simulink model "ramadan_2021"  (R2020a)
settings: Solver=ode15s  StartTime=0.0  StopTime=20  MaxStep=1e-2  MinStep=1e-20  RelTol=1e-3
StartFcn:
  | tic
StopFcn:
  | toc
  | 
  | 
  | %if GimbalLockFlag
  |  % fprintf(2, 'Almost reached Gimbal Lock of IMU. Simulation stopped.\n')
  | %end
  | 
  | %fprintf('Elapsed time: %4.2f sec (%4.2f%% realtime)\n', a, tout(end)/a*100)
values from neighbouring files (symbols this model uses):
  Balance02 = param(28:31)    [assign_parameters.m]
  Balance13 = param(32:35)    [assign_parameters.m]
  BalanceTrunk = param(22:23)    [assign_parameters.m]
  BalanceTrunkLat = param(24:27)    [assign_parameters.m]
  BasisStim = param(1:11)    [assign_parameters.m]
  CompliantLeg = param(12:14)    [assign_parameters.m]
  CompliantLegLat = param(15)    [assign_parameters.m]
  PreventKneeOverextension = param(16:21)    [assign_parameters.m]
  propulsion = dataset(i,3)    [AssignDataset_BasisPoints.m]    (also in assign_parameters.m = param(43))
  stepDur = dataset(i,2)    [AssignDataset_BasisPoints.m]    (also in assign_parameters.m = param(44))
  Target02 = dataset(i,8:10)    [AssignDataset_BasisPoints.m]    (also in assign_parameters.m = param(36:38))
  Target13 = dataset(i,5:7)    [AssignDataset_BasisPoints.m]    (also in assign_parameters.m = param(39:41))
  Target_lat = param(45)    [assign_parameters.m]
  theta0 = dataset(i,4)    [AssignDataset_BasisPoints.m]    (also in assign_parameters.m = param(42))
  v_init = dataset(i,1)    [AssignDataset_BasisPoints.m]    (also in assign_parameters.m = 1.25)
  WramameiSL_1000 = readmatrix('WSL_1000_Norm_Sigmoid_MSE_cont.csv')    [nms3D_prep.m]
  ZramameiSL_1000 = readmatrix('ZSL_1000_Norm_Sigmoid_MSE_cont.csv')    [nms3D_prep.m]
undefined symbols (not defined in the file or in its folder): ICs, mParams, X, Y, Z
libraries: nesl_utility x110, sm_lib x88, simulink x81, eeGeneralControl x30, robotmaniplib x10, dspinverses x9, robotcorelib x5, dspmathops x3, vrlib x1
(part 7 of 8)

== system ramadan_2021/Muscle Actuation Layer/Muscles Right/Muscle Dynamics (Vectorized)/CE inverse force-velocity relation ==
  note: CE Inverse Force-Velocity Relationship
  Fv[Fmax] : Inport
  1 : Product  Inputs=/*
  Constant{1,3..4,8} (4 alike) : Constant
  Constant2 : Constant  Value=mParams.muscles.N
  Curvature : Gain  Gain=mParams.muscles.K  SaturateOnIntegerOverflow=on  OutDataTypeStr=Inherit: Same as input  ParamDataTypeStr=Inherit: Same as input
  Curvature1 : Gain  Gain=7.56*mParams.muscles.K  SaturateOnIntegerOverflow=on  OutDataTypeStr=Inherit: Same as input  ParamDataTypeStr=Inherit: Same as input
  Logical Operator : Logic  Operator=NOT  AllPortsSameDT=off  OutDataTypeStr=boolean
  Logical Operator1 : Logic  Operator=NOT  AllPortsSameDT=off  OutDataTypeStr=boolean
  Slope : Gain  Gain=1e-2  SaturateOnIntegerOverflow=on  OutDataTypeStr=Inherit: Same as input  ParamDataTypeStr=Inherit: Same as input
  Sum1 : Sum  Inputs=|++  InputSameDT=on  SaturateOnIntegerOverflow=on  OutDataTypeStr=Inherit: Same as first input
  Sum2 : Sum  InputSameDT=on  SaturateOnIntegerOverflow=on  OutDataTypeStr=Inherit: Same as first input
  Sum3 : Sum  Inputs=++|  InputSameDT=on  SaturateOnIntegerOverflow=on  OutDataTypeStr=Inherit: Same as first input
  Sum4 : Sum  Inputs=|+-  InputSameDT=on  SaturateOnIntegerOverflow=on  OutDataTypeStr=Inherit: Same as first input
  Sum5 : Sum  Inputs=|-+  InputSameDT=on  SaturateOnIntegerOverflow=on  OutDataTypeStr=Inherit: Same as first input
  Sum6 : Sum  Inputs=-+|  InputSameDT=on  SaturateOnIntegerOverflow=on  OutDataTypeStr=Inherit: Same as first input
  Sum7 : Sum  Inputs=|++  InputSameDT=on  SaturateOnIntegerOverflow=on  OutDataTypeStr=Inherit: Same as first input
  Sum8 : Sum  Inputs=+-|  InputSameDT=on  SaturateOnIntegerOverflow=on  OutDataTypeStr=Inherit: Same as first input
  Sum9 : Sum  InputSameDT=on  SaturateOnIntegerOverflow=on  OutDataTypeStr=Inherit: Same as first input
  extension force within bound? : simulink/Logic and Bit Operations/Compare To Constant  relop=<=  const=mParams.muscles.N  OutDataTypeStr=boolean  ZeroCross=off
  force indicating contraction? : simulink/Logic and Bit Operations/Compare To Constant  relop=<=  const=1  OutDataTypeStr=boolean  ZeroCross=off
  v_concentric : Product  Inputs=*/
  v_concentric1 : Product  Inputs=**
  v_excentric <=N 1 : Product  Inputs=***
  v_excentric <N : Product  Inputs=*/
  v_excentric >N : Product  Inputs=**
  v[vmax] : Outport  VectorParamsAs1DForOutWhenUnconnected=off
  wires:
  Sum2/1 -> Sum9/2
  v_excentric <=N 1/1 -> Sum2/1
  Logical Operator1/1 -> v_excentric >N/1
  v_excentric >N/1 -> Sum2/2
  Logical Operator/1 -> v_excentric <=N 1/1
  Fv[Fmax]/1 -> extension force within bound?/1, force indicating contraction?/1, Curvature/1, Sum4/1, Sum6/2
  extension force within bound?/1 -> Logical Operator1/1, v_excentric <=N 1/3
  force indicating contraction?/1 -> Logical Operator/1, v_concentric1/2
  Sum1/1 -> v_excentric >N/2
  v_concentric1/1 -> Sum9/1
  v_excentric <N/1 -> v_excentric <=N 1/2
  Constant3/1 -> Sum5/1
  Sum5/1 -> 1/1
  Constant2/1 -> Sum5/2, Sum6/1
  Sum6/1 -> Slope/1, 1/2
  Constant8/1 -> Sum1/2
  Slope/1 -> Sum1/1
  Sum9/1 -> v[vmax]/1
  v_concentric/1 -> v_concentric1/1
  Sum7/1 -> v_excentric <N/1
  Sum8/1 -> v_excentric <N/2
  Curvature1/1 -> Sum8/2
  Constant4/1 -> Sum8/1, Sum7/2
  1/1 -> Curvature1/1, Sum7/1
  Sum3/1 -> v_concentric/2
  Sum4/1 -> v_concentric/1
  Constant1/1 -> Sum3/1, Sum4/2
  Curvature/1 -> Sum3/2

== system ramadan_2021/Muscle Actuation Layer/Muscles Right/Muscle Dynamics (Vectorized)/PE force-length relation ==
  note: Parallel Elasticity PE
  lce [lopt] : Inport
  Constant3 : Constant
  Math Function2 : Math  Operator=square  SignedPower=on  SaturateOnIntegerOverflow=on
  Sum1 : Sum  Inputs=|+-  InputSameDT=on  SaturateOnIntegerOverflow=on  OutDataTypeStr=Inherit: Same as first input
  force of buffer elasticity : Product  Inputs=**
  parallel elasticity engaged? : simulink/Logic and Bit Operations/Compare To Zero  relop=>  OutDataTypeStr=boolean  ZeroCross=off
  reference strain [lopt] : Constant  Value=mParams.muscles.w
  relative strain : Product  Inputs=*/
  fpe [Fmax] : Outport  VectorParamsAs1DForOutWhenUnconnected=off
  wires:
  parallel elasticity engaged?/1 -> force of buffer elasticity/1
  force of buffer elasticity/1 -> fpe [Fmax]/1
  Math Function2/1 -> force of buffer elasticity/2
  relative strain/1 -> Math Function2/1
  reference strain [lopt]/1 -> relative strain/2
  Sum1/1 -> relative strain/1, parallel elasticity engaged?/1
  Constant3/1 -> Sum1/2
  lce [lopt]/1 -> Sum1/1

== system ramadan_2021/Muscle Actuation Layer/Muscles Right/Muscle Dynamics (Vectorized)/SE force-length relation ==
  note: SE Force-Length Relationship
  lse [lslack] : Inport
  Constant1 : Constant
  Math Function : Math  Operator=square  SignedPower=on  SaturateOnIntegerOverflow=on
  Sum4 : Sum  Inputs=|+-  InputSameDT=on  SaturateOnIntegerOverflow=on  OutDataTypeStr=Inherit: Same as first input
  force above slack length : Product  Inputs=**
  greater than slack length? : simulink/Logic and Bit Operations/Compare To Zero  relop=>  OutDataTypeStr=boolean  ZeroCross=off
  reference strain [lslack] : Constant  Value=mParams.muscles.eref
  relative strain : Product  Inputs=*/
  fse [Fmax] : Outport  VectorParamsAs1DForOutWhenUnconnected=off
  wires:
  force above slack length/1 -> fse [Fmax]/1
  greater than slack length?/1 -> force above slack length/1
  Constant1/1 -> Sum4/2
  Sum4/1 -> relative strain/1, greater than slack length?/1
  relative strain/1 -> Math Function/1
  lse [lslack]/1 -> Sum4/1
  Math Function/1 -> force above slack length/2
  reference strain [lslack]/1 -> relative strain/2

== system ramadan_2021/Muscle Actuation Layer/Muscles Right/Muscle Torque Contributions/Subsystem ==
  F VAS : Inport
  Moment Arm VAS : Inport  Port=2
  F SOL : Inport  Port=3
  Moment Arm SOL : Inport  Port=4
  Constant : Constant  Value=mParams.muscles.FmaxVec(7)
  Constant1 : Constant  Value=mParams.muscles.FmaxVec(10)
  Divide2 : Product  Inputs=*/
  Product{7..8,11..12} (4 alike) : Product
  Sum4 : Sum
  Sum6 : Sum
  "Leg Torque " : Outport
  wires:
  Sum4/1 -> Divide2/2
  Divide2/1 -> "Leg Torque "/1
  Moment Arm SOL/1 -> Product7/1, Product11/2
  Product11/1 -> Sum6/2
  Constant/1 -> Product8/2
  F VAS/1 -> Product12/1
  Moment Arm VAS/1 -> Product8/1, Product12/2
  Product7/1 -> Sum4/2
  F SOL/1 -> Product11/1
  Sum6/1 -> Divide2/1
  Product12/1 -> Sum6/1
  Constant1/1 -> Product7/2
  Product8/1 -> Sum4/1

== system ramadan_2021/Supraspinal Level/Subsystem/Compute positives forces that generate desired torque profiles/Left ==
  Desired Torques : Inport
  Angles : Inport  Port=2
  Constant : Constant  Value=WramameiSL_1000  VectorParams1D=off  SampleTime=-1
  Constant1 : Constant  Value=|
      | [1.666708374023437500e+01
      | -3.333266830444335938e+01]
  Constant2 : Constant  Value=ZramameiSL_1000
  Denorm : Gain  Gain=[2000, 1500, 3000, 1200, 6000, 350, 1500, 4000, 800]
  Matrix Concatenate : Concatenate  Mode=Multidimensional array
  Matrix Concatenate4 : Concatenate  Mode=Multidimensional array  ConcatenateDimension=2
  Matrix Multiply2 : Product  Multiplication=Matrix(*)
  Matrix Multiply3 : Product  Multiplication=Matrix(*)
  Matrix Multiply8 : Product  Multiplication=Matrix(*)
  Multiply : Gain  Gain=1/960
  Multiply2 : Gain  Gain=1/3.0543
  Saturation : Saturate  UpperLimit=inf  LowerLimit=0  ZeroCross=off
  Saturation2 : Saturate  UpperLimit=inf  LowerLimit=0  ZeroCross=off
  Selector : Selector  InputPortWidth=4  IndexOptions=Index vector (dialog)  Indices=[1 3 4]  OutputSizes=1
  Selector1 : Selector  InputPortWidth=4  IndexOptions=Index vector (dialog)  Indices=[3 4]  OutputSizes=1
  Selector8 : Selector  InputPortWidth=4  IndexOptions=Index vector (dialog)  Indices=2  OutputSizes=1
  Transpose3 : Math  Operator=transpose  SaturateOnIntegerOverflow=on
  Transpose9 : Math  Operator=transpose  SaturateOnIntegerOverflow=on
  sigmoid : Subsystem
  Forces : Outport
  wires:
  Desired Torques/1 -> Selector/1, Selector8/1
  Selector1/1 -> Multiply2/1
  Matrix Multiply2/1 -> Saturation/1
  Selector/1 -> Multiply/1
  Constant/1 -> Matrix Multiply3/2
  Constant2/1 -> Matrix Multiply2/2
  Angles/1 -> Selector1/1
  Matrix Multiply8/1 -> Saturation2/1
  Constant1/1 -> Transpose9/1
  Selector8/1 -> Matrix Multiply8/1
  Transpose9/1 -> Matrix Multiply8/2
  Saturation/1 -> Denorm/1
  Matrix Concatenate4/1 -> Forces/1
  Saturation2/1 -> Matrix Concatenate4/1
  Transpose3/1 -> Matrix Multiply3/1
  Matrix Concatenate/1 -> Transpose3/1  "tr"
  Denorm/1 -> Matrix Concatenate4/2
  Multiply/1 -> Matrix Concatenate/1
  Multiply2/1 -> Matrix Concatenate/2
  sigmoid/1(Out1) -> Matrix Multiply2/1
  Matrix Multiply3/1 -> sigmoid/1(In1)

== system ramadan_2021/Supraspinal Level/Subsystem/Compute positives forces that generate desired torque profiles/Right ==
  Desired Torques : Inport
  Angles : Inport  Port=2
  Constant : Constant  Value=WramameiSL_1000  VectorParams1D=off  SampleTime=-1
  Constant1 : Constant  Value=|
      | [1.666708374023437500e+01
      | -3.333266830444335938e+01]
  Constant2 : Constant  Value=ZramameiSL_1000
  Denorm : Gain  Gain=[2000, 1500, 3000, 1200, 6000, 350, 1500, 4000, 800]
  Matrix Concatenate : Concatenate  Mode=Multidimensional array
  Matrix Concatenate4 : Concatenate  Mode=Multidimensional array  ConcatenateDimension=2
  Matrix Multiply2 : Product  Multiplication=Matrix(*)
  Matrix Multiply3 : Product  Multiplication=Matrix(*)
  Matrix Multiply8 : Product  Multiplication=Matrix(*)
  Multiply : Gain  Gain=1/960
  Multiply2 : Gain  Gain=1/3.0543
  Saturation : Saturate  UpperLimit=inf  LowerLimit=0  ZeroCross=off
  Saturation2 : Saturate  UpperLimit=inf  LowerLimit=0  ZeroCross=off
  Selector : Selector  InputPortWidth=4  IndexOptions=Index vector (dialog)  Indices=[1 3 4]  OutputSizes=1
  Selector1 : Selector  InputPortWidth=4  IndexOptions=Index vector (dialog)  Indices=[3 4]  OutputSizes=1
  Selector8 : Selector  InputPortWidth=4  IndexOptions=Index vector (dialog)  Indices=2  OutputSizes=1
  Transpose3 : Math  Operator=transpose  SaturateOnIntegerOverflow=on
  Transpose9 : Math  Operator=transpose  SaturateOnIntegerOverflow=on
  sigmoid : Subsystem
  Forces : Outport
  wires:
  Desired Torques/1 -> Selector/1, Selector8/1
  Selector1/1 -> Multiply2/1
  Matrix Multiply2/1 -> Saturation/1
  Selector/1 -> Multiply/1
  Constant/1 -> Matrix Multiply3/2
  Constant2/1 -> Matrix Multiply2/2
  Angles/1 -> Selector1/1
  Matrix Multiply8/1 -> Saturation2/1
  Constant1/1 -> Transpose9/1
  Selector8/1 -> Matrix Multiply8/1
  Transpose9/1 -> Matrix Multiply8/2
  Saturation/1 -> Denorm/1
  Matrix Concatenate4/1 -> Forces/1
  Saturation2/1 -> Matrix Concatenate4/1
  Transpose3/1 -> Matrix Multiply3/1
  Matrix Concatenate/1 -> Transpose3/1  "tr"
  Denorm/1 -> Matrix Concatenate4/2
  Multiply/1 -> Matrix Concatenate/1
  Multiply2/1 -> Matrix Concatenate/2
  sigmoid/1(Out1) -> Matrix Multiply2/1
  Matrix Multiply3/1 -> sigmoid/1(In1)

== system ramadan_2021/Supraspinal Level/Subsystem/Stance Leg2/Balance Control Equation [Ankle Strategy] ==
  Desired Acceleration (CoM) : Outport
  wires:
  [propulsion] -> Desired Acceleration (CoM)/1

== system ramadan_2021/Supraspinal Level/Subsystem/Stance Leg2/Stance Leg ==
  left/right : Inport
  Balance Control [Ankle Strategy] : Inport  Port=2
  Foot Orientation Left : Subsystem
  Foot Orientation Right : Subsystem
  Inverse Dynamics Left Leg : Subsystem
  Mux : Mux  Inputs=2
  Mux1 : Mux  Inputs=2
  NOT2 : Logic  Operator=NOT  AllPortsSameDT=off  OutDataTypeStr=boolean
  Selector : Selector  InputPortWidth=4  IndexOptions=Index vector (dialog)  Indices=[ 4 3 2 1]  OutputSizes=1
  Selector1 : Selector  InputPortWidth=4  IndexOptions=Index vector (dialog)  Indices=[ 4 3 2 1]  OutputSizes=1
  Subsystem : Subsystem
  Transpose : Math  Operator=transpose  SaturateOnIntegerOverflow=on
  long delay 1 : eeGeneralControl/Low-Pass Filter (Discrete or Continuous)  K=1  T=mParams.control.delays.long  B=inf  A=-inf  init_option=Inherited from block input  x0=0  Ts=0
  long delay 2 : eeGeneralControl/Low-Pass Filter (Discrete or Continuous)  K=1  T=mParams.control.delays.long  B=inf  A=-inf  init_option=Inherited from block input  x0=0  Ts=0
  long delay 4 : eeGeneralControl/Low-Pass Filter (Discrete or Continuous)  K=1  T=mParams.control.delays.long  B=inf  A=-inf  init_option=Inherited from block input  x0=0  Ts=0
  Push Off Left : Outport
  Push-Off Right : Outport  Port=2
  wires:
  [Rlegq] -> long delay 2/1
  Selector/1 -> Mux/2
  Selector1/1 -> Mux1/2
  [R_body] -> long delay 4/1
  left/right/1 -> NOT2/1, Inverse Dynamics Left Leg/2(left/right)
  Transpose/1 -> Foot Orientation Right/1(R Pelvis), Foot Orientation Left/1(R Pelvis)
  Foot Orientation Left/1(Orientation Foot (Z)) -> Mux1/1
  Foot Orientation Right/1(Foot Orientation (Z)) -> Mux/1
  Balance Control [Ankle Strategy]/1 -> Inverse Dynamics Left Leg/3(Task), Subsystem/3(Task)
  Inverse Dynamics Left Leg/1(Push-Off (Left)) -> Push Off Left/1
  Mux/1 -> Subsystem/1(Config [5])
  NOT2/1 -> Subsystem/2(left/right)
  Subsystem/1(Push-Off (Right)) -> Push-Off Right/1
  Mux1/1 -> Inverse Dynamics Left Leg/1(Config [5])
  long delay 1/1 -> Selector1/1
  long delay 2/1 -> Selector/1
  long delay 4/1 -> Transpose/1
  [Llegq] -> long delay 1/1

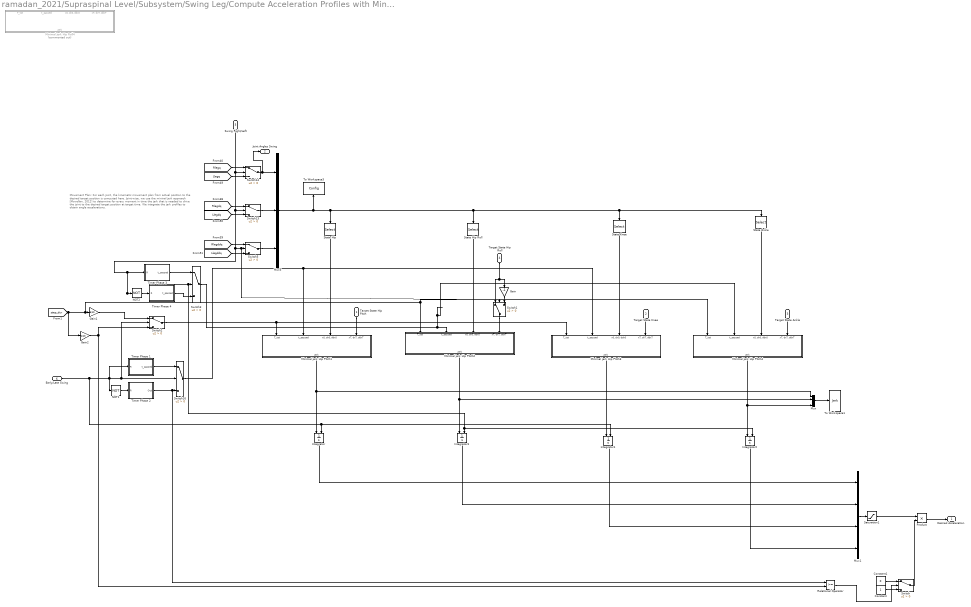
== system ramadan_2021/Supraspinal Level/Subsystem/Swing Leg/Compute Acceleration Profiles with Minimal Jerk Approach ==
  note: Movement Plan: For each joint, the kinematic movement plan from actual position to the desired target position is computed here. Joint-wise, we use the mininal jerk approach [Movellan, 2012] to determine for every moment in time the jerk that is needed to drive the joint to the desired target position at target time. We integrate the jerk profiles to obtain angle accelerations.
  Target State Hip Pitch : Inport
  Target State Knee : Inport  Port=2
  Target State Ankle : Inport  Port=3
  Target State Hip Roll : Inport  Port=4
  Swing Right/Left : Inport  Port=5
  Early/Late Swing : Inport  Port=6
  " Timer Phase 1" : Subsystem
  " Timer Phase 2" : Subsystem
  " Timer Phase 3" : Subsystem
  " Timer Phase 4" : Subsystem
  Constant : Constant
  Constant1 : Constant  Value=0
  Gain : Gain  Gain=-1
  Gain1 : Gain  Gain=6/10
  Gain2 : Gain  Gain=4/10
  Integrator{,1..3} (4 alike) : Integrator  ExternalReset=either  ZeroCross=off
  Minimal jerk Hip Pitch1 : Subsystem
  Minimal jerk Hip Pitch2 : Subsystem
  Minimal jerk Hip Pitch3 : Subsystem
  Minimal jerk Hip Pitch4 : Subsystem
  Minimal jerk Hip Roll4 : Subsystem  Commented=on
  Mux : Mux
  Mux1 : Mux
  Mux5 : Mux  Inputs=3
  NOT1 : Logic  Operator=NOT  AllPortsSameDT=off  OutDataTypeStr=boolean
  NOT2 : Logic  Operator=NOT  AllPortsSameDT=off  OutDataTypeStr=boolean
  Product : Product
  Relational Operator : RelationalOperator  OutDataTypeStr=boolean  ZeroCross=off  RndMeth=Simplest
  Saturation1 : Saturate  UpperLimit=2000  LowerLimit=-2000  ZeroCross=off
  State Ankle : Selector  InputPortWidth=12  IndexOptions=Index vector (dialog)  Indices=[4 8 12]  OutputSizes=1
  State Hip : Selector  InputPortWidth=12  IndexOptions=Index vector (dialog)  Indices=[1 5 9]  OutputSizes=1
  State Hip Roll : Selector  InputPortWidth=12  IndexOptions=Index vector (dialog)  Indices=[2 6 10 ]  OutputSizes=1
  State Knee : Selector  InputPortWidth=12  IndexOptions=Index vector (dialog)  Indices=[3 7 11 ]  OutputSizes=1
  Switch{,1..3,5,13..14,16} (8 alike) : Switch  Criteria=u2 > Threshold
  To Workspace1 : ToWorkspace  VariableName=Jerk  SampleTime=-1
      settings: Save2DSignal=2-D array (concatenate along first dimension)
  To Workspace3 : ToWorkspace  VariableName=Config  SampleTime=-1
      settings: Save2DSignal=2-D array (concatenate along first dimension)
  "Desired Acceleration " : Outport
  Joint Angles Swing : Outport  Port=2
  wires:
  State Hip/1 -> Minimal jerk Hip Pitch1/3("x0, dx0, ddx0")
  NOT1/1 -> " Timer Phase 2"/1(R)
  Mux1/1 -> Saturation1/1
  Switch2/1 -> Minimal jerk Hip Pitch1/1(T_tot), Minimal jerk Hip Pitch3/1(T_tot)
  [Llegddq] -> Switch5/3
  [Rlegq] -> Switch14/1
  [Llegdq] -> Switch13/3
  Target State Hip Pitch/1 -> Minimal jerk Hip Pitch1/4("xT, dxT, ddxT")
  Target State Knee/1 -> Minimal jerk Hip Pitch3/4("xT, dxT, ddxT")
  [Rlegddq] -> Switch5/1
  Integrator1/1 -> Mux1/3
  Switch5/1 -> Mux5/3
  [Llegq] -> Switch14/3
  State Knee/1 -> Minimal jerk Hip Pitch3/3("x0, dx0, ddx0")
  Target State Ankle/1 -> Minimal jerk Hip Pitch4/4("xT, dxT, ddxT")
  Integrator/1 -> Mux1/1
  Switch14/1 -> Joint Angles Swing/1, Mux5/1
  Integrator2/1 -> Mux1/4
  State Ankle/1 -> Minimal jerk Hip Pitch4/3("x0, dx0, ddx0")
  Switch13/1 -> Mux5/2
  [Rlegdq] -> Switch13/1
  Early/Late Swing/1 -> Switch2/2, Switch16/2, NOT1/1, " Timer Phase 1"/1(R), Integrator1/2, Integrator/2
  Swing Right/Left/1 -> Switch14/2, Switch13/2, Integrator2/2, Integrator3/2, Switch3/2, NOT2/1, " Timer Phase 3"/1(R), Switch1/2, Switch5/2
  Switch16/1 -> Minimal jerk Hip Pitch1/2(t_passed), Minimal jerk Hip Pitch3/2(t_passed)
  State Hip Roll/1 -> Minimal jerk Hip Pitch2/3("x0, dx0, ddx0")
  Integrator3/1 -> Mux1/2
  Switch1/1 -> Minimal jerk Hip Pitch2/4("xT, dxT, ddxT")
  Target State Hip Roll/1 -> Gain/1, Switch1/1
  Gain/1 -> Switch1/3
  [step_dur] -> Gain2/1, Minimal jerk Hip Pitch4/1(T_tot), Minimal jerk Hip Pitch2/1(T_tot), Gain1/1
  " Timer Phase 1"/1(t_passed) -> Switch16/1
  " Timer Phase 2"/1(Out) -> Relational Operator/1, Switch16/3
  Mux5/1 -> State Hip Roll/1, State Ankle/1, State Knee/1, State Hip/1, To Workspace3/1
  Mux/1 -> To Workspace1/1
  Minimal jerk Hip Pitch1/1(jerk) -> Mux/1, Integrator/1
  Minimal jerk Hip Pitch2/1(jerk) -> Mux/2, Integrator3/1
  Minimal jerk Hip Pitch3/1(jerk) -> Integrator1/1
  Minimal jerk Hip Pitch4/1(jerk) -> Mux/4, Integrator2/1
  Saturation1/1 -> Product/1
  Relational Operator/1 -> Switch/2
  Constant/1 -> Switch/3
  Constant1/1 -> Switch/1
  Switch/1 -> Product/2
  Product/1 -> "Desired Acceleration "/1
  Gain1/1 -> Switch2/1
  Gain2/1 -> Switch2/3, Relational Operator/2
  NOT2/1 -> " Timer Phase 4"/1(R)
  " Timer Phase 3"/1(t_passed) -> Switch3/1
  " Timer Phase 4"/1(t_passed) -> Switch3/3
  Switch3/1 -> Minimal jerk Hip Pitch4/2(t_passed), Minimal jerk Hip Pitch2/2(t_passed)

== system ramadan_2021/Supraspinal Level/Subsystem/Swing Leg/Compute Target States ==
  note: Target Joint States: Target joint angles, angle velocities and angle acceleration are defined here. For knee and ankle, values are constant. For hip pitch and hip roll, values are computed using the Balance Control mechanism from [Yin et. al. 2007].
      | Low pass filters are added here to compensate for abrupt changes in target angles at transitions between early and late swing.
  Left/Right : Inport
  Early/Late : Inport  Port=2
  Balance Control lateral : Subsystem
  Balance Control saggital : Subsystem
  Constant : Constant  Value=0
  Constant13 : Constant  Value=pi
  Gain3 : Gain  Gain=-1
  Low-Pass Filter (Discrete or Continuous)1 : eeGeneralControl/Low-Pass Filter (Discrete or Continuous)  K=1  T=0.1  B=inf  A=-inf  init_option=Inherited from block input  x0=-13  Ts=0
  Low-Pass Filter (Discrete or Continuous)2 : eeGeneralControl/Low-Pass Filter (Discrete or Continuous)  K=1  T=0.1  B=inf  A=-inf  init_option=Inherited from block input  x0=-13  Ts=0
  Minus1 : Sum
  Minus8 : Sum  Inputs=+++
  Mux{2..3,5..6} (4 alike) : Mux  Inputs=3
  Product : Product
  Sign : Signum  ZeroCross=off
  Hip Pitch Target : Outport
  Knee Target : Outport  Port=2
  Ankle Target : Outport  Port=3
  Hip Roll Target : Outport  Port=4
  wires:
  [TrunkRot_sag] -> Minus8/3
  Left/Right/1 -> Balance Control lateral/1(Left/Right), Balance Control saggital/1(Left/Right)
  Gain3/1 -> Minus8/1
  [swk] -> Mux5/1
  Balance Control lateral/1(theta_Hip_swing_target) -> Sign/1, Minus1/1
  Balance Control saggital/1(theta_Hip_swing_target) -> Gain3/1
  Mux5/1 -> Knee Target/1
  Constant13/1 -> Minus8/2
  [TrunkRot_lat] -> Minus1/2
  Mux2/1 -> Low-Pass Filter (Discrete or Continuous)2/1
  Mux6/1 -> Ankle Target/1
  Minus1/1 -> Mux2/1
  Low-Pass Filter (Discrete or Continuous)2/1 -> Hip Roll Target/1
  [swa] -> Mux6/1
  [swh_lat_a] -> Mux2/3
  [swh_lat_v] -> Product/1
  Product/1 -> Mux2/2
  Sign/1 -> Product/2
  Minus8/1 -> Mux3/1
  Mux3/1 -> Low-Pass Filter (Discrete or Continuous)1/1
  Low-Pass Filter (Discrete or Continuous)1/1 -> Hip Pitch Target/1
  Early/Late/1 -> Balance Control saggital/2(Early Late)
  Constant/1 -> Mux6/3, Mux6/2, Mux5/3, Mux3/2, Mux3/3, Mux5/2

== system ramadan_2021/Supraspinal Level/Subsystem/Swing Leg/Inverse Dynamics: Left Leg ==
  Desired Acceleration : Inport
  Enable : Inport  Port=2
  Inverse Dynamics : Subsystem
  Sensor Data from Body Layer : Subsystem
  Desired Torques : Outport
  Interaction Wrench : Outport  Port=2
  wires:
  Inverse Dynamics/1(" Desired Torques") -> Desired Torques/1
  Desired Acceleration/1 -> Inverse Dynamics/8(Desired Acceleration [rad/s^2])
  Sensor Data from Body Layer/4(" Rotation Trunk [rad]") -> Inverse Dynamics/4(Rotation Trunk [rad])
  Sensor Data from Body Layer/2(Joint Angle Velocities [rad/s]) -> Inverse Dynamics/2(Joint Angle Velocities [rad/s])
  Sensor Data from Body Layer/1(Joint Angles [rad]) -> Inverse Dynamics/1(Joint Angles [rad])
  Sensor Data from Body Layer/6(Rotation Velocity Trunk [rad/s]) -> Inverse Dynamics/6(Rotation Velocity Trunk [rad/s])
  Sensor Data from Body Layer/5(Trunk Position [m]) -> Inverse Dynamics/5(Trunk Position [m])
  Sensor Data from Body Layer/7(Trunk Velocity [m/s]) -> Inverse Dynamics/7(Trunk Velocity [m/s])
  Enable/1 -> Inverse Dynamics/Enable
  Inverse Dynamics/2(Interaction Wrench) -> Interaction Wrench/1
  Sensor Data from Body Layer/3(Joint Angle Accelerations [rad/s^2]) -> Inverse Dynamics/3(Joint  Acceleration [rad/s^2])

== system ramadan_2021/Supraspinal Level/Subsystem/Swing Leg/Inverse Dynamics: Right Leg ==
  Desired Acceleration : Inport
  Enable : Inport  Port=2
  Inverse Dynamics1 : Subsystem
  Sensor Data from Body Layer1 : Subsystem
  Desired Torques : Outport
  Interaction Wrench : Outport  Port=2
  wires:
  Inverse Dynamics1/1(" Desired Torques") -> Desired Torques/1
  Enable/1 -> Inverse Dynamics1/Enable
  Inverse Dynamics1/2(Interaction Wrench) -> Interaction Wrench/1
  Sensor Data from Body Layer1/1(Joint Angles [rad]) -> Inverse Dynamics1/1(Joint Angles [rad])
  Sensor Data from Body Layer1/2(Joint Angle Velocities [rad/s]) -> Inverse Dynamics1/2(Joint Angle Velocities [rad/s])
  Sensor Data from Body Layer1/3(Joint Angle Accelerations [rad/s^2]) -> Inverse Dynamics1/3(Joint  Acceleration [rad/s^2])
  Sensor Data from Body Layer1/4(" Rotation Trunk [rad]") -> Inverse Dynamics1/4(Rotation Trunk [rad])
  Sensor Data from Body Layer1/5(Trunk Position [m]) -> Inverse Dynamics1/5(Trunk Position [m])
  Sensor Data from Body Layer1/6(Rotation Velocity Trunk [rad/s]) -> Inverse Dynamics1/6(Rotation Velocity Trunk [rad/s])
  Sensor Data from Body Layer1/7(Trunk Velocity [m/s]) -> Inverse Dynamics1/7(Trunk Velocity [m/s])
  Desired Acceleration/1 -> Inverse Dynamics1/8(Desired Acceleration [rad/s^2])

== system ramadan_2021/Supraspinal Level/Subsystem/Compute positives forces that generate desired torque profiles/Left/sigmoid ==
  In1 : Inport
  Add : Sum
  Constant : Constant
  Constant1 : Constant
  Divide : Product  Inputs=*/
  Exp : Math  SaturateOnIntegerOverflow=on
  Gain : Gain  Gain=-1
  Out1 : Outport
  wires:
  Constant/1 -> Divide/1
  Constant1/1 -> Add/1
  In1/1 -> Gain/1
  Gain/1 -> Exp/1
  Exp/1 -> Add/2
  Add/1 -> Divide/2
  Divide/1 -> Out1/1

== system ramadan_2021/Supraspinal Level/Subsystem/Compute positives forces that generate desired torque profiles/Right/sigmoid ==
  In1 : Inport
  Add : Sum
  Constant : Constant
  Constant1 : Constant
  Divide : Product  Inputs=*/
  Exp : Math  SaturateOnIntegerOverflow=on
  Gain : Gain  Gain=-1
  Out1 : Outport
  wires:
  Constant/1 -> Divide/1
  Constant1/1 -> Add/1
  In1/1 -> Gain/1
  Gain/1 -> Exp/1
  Exp/1 -> Add/2
  Add/1 -> Divide/2
  Divide/1 -> Out1/1

== system ramadan_2021/Supraspinal Level/Subsystem/Stance Leg2/Stance Leg/Foot Orientation Left ==
  R Pelvis : Inport
  Coordinate Transformation Conversion1 : robotcorelib/Coordinate Transformation Conversion  InputRepresentation=Rotation Matrix  InputEulerSequence=ZYX  ShowTrVecInputPort=on  OutputRepresentation=Euler Angles  OutputEulerSequence=XYZ  ShowTrVecOutputPort=on  SimulateUsing=Code generation
      settings: SourceProductBaseCode=NV,RO,RR
  Matrix Multiply : Product  Multiplication=Matrix(*)
  Selector2 : Selector  InputPortWidth=3  IndexOptions=Index vector (dialog)  Indices=[ 3]  OutputSizes=1
  Orientation Foot (Z) : Outport
  wires:
  Coordinate Transformation Conversion1/1 -> Selector2/1
  Matrix Multiply/1 -> Coordinate Transformation Conversion1/1
  Selector2/1 -> Orientation Foot (Z)/1
  R Pelvis/1 -> Matrix Multiply/1
  [RotationMatrixLeftFoot] -> Matrix Multiply/2

== system ramadan_2021/Supraspinal Level/Subsystem/Stance Leg2/Stance Leg/Foot Orientation Right ==
  R Pelvis : Inport
  Coordinate Transformation Conversion3 : robotcorelib/Coordinate Transformation Conversion  InputRepresentation=Rotation Matrix  InputEulerSequence=ZYX  ShowTrVecInputPort=on  OutputRepresentation=Euler Angles  OutputEulerSequence=XYZ  ShowTrVecOutputPort=on  SimulateUsing=Code generation
      settings: SourceProductBaseCode=NV,RO,RR
  Matrix Multiply1 : Product  Multiplication=Matrix(*)
  Selector3 : Selector  InputPortWidth=3  IndexOptions=Index vector (dialog)  Indices=[ 3]  OutputSizes=1
  Foot Orientation (Z) : Outport
  wires:
  R Pelvis/1 -> Matrix Multiply1/1
  Selector3/1 -> Foot Orientation (Z)/1
  Coordinate Transformation Conversion3/1 -> Selector3/1
  [RotationMatrixRightFoot] -> Matrix Multiply1/2
  Matrix Multiply1/1 -> Coordinate Transformation Conversion3/1

== system ramadan_2021/Supraspinal Level/Subsystem/Stance Leg2/Stance Leg/Inverse Dynamics Left Leg ==
  Config [5] : Inport
  left/right : Inport  Port=2
  Task : Inport  Port=3
  Left Leg Ball : Subsystem
  Low-Pass Filter (Discrete or Continuous) : eeGeneralControl/Low-Pass Filter (Discrete or Continuous)  K=1  T=0.01  B=150  A=-150  init_option=Inherited from block input  x0=0  Ts=0
  Product : Product
  Selector4 : Selector  InputPortWidth=5  IndexOptions=Index vector (dialog)  Indices=[ 5 4 3 2]  OutputSizes=1
  Push-Off (Left) : Outport
  wires:
  Product/1 -> Selector4/1
  Selector4/1 -> Low-Pass Filter (Discrete or Continuous)/1
  Left Leg Ball/1(Push-Off Left (Ball)) -> Product/1
  Task/1 -> Left Leg Ball/2(Task)
  left/right/1 -> Product/2, Left Leg Ball/Enable
  Low-Pass Filter (Discrete or Continuous)/1 -> Push-Off (Left)/1
  Config [5]/1 -> Left Leg Ball/1(Config)

== system ramadan_2021/Supraspinal Level/Subsystem/Stance Leg2/Stance Leg/Subsystem ==
  Config [5] : Inport
  left/right : Inport  Port=2
  Task : Inport  Port=3
  Low-Pass Filter (Discrete or Continuous)1 : eeGeneralControl/Low-Pass Filter (Discrete or Continuous)  K=1  T=0.01  B=150  A=-150  init_option=Inherited from block input  x0=0  Ts=0
  Product1 : Product
  Right Leg Ball : Subsystem
  Selector5 : Selector  InputPortWidth=5  IndexOptions=Index vector (dialog)  Indices=[ 5 4 3 2]  OutputSizes=1
  Push-Off (Right) : Outport
  wires:
  Selector5/1 -> Low-Pass Filter (Discrete or Continuous)1/1
  Low-Pass Filter (Discrete or Continuous)1/1 -> Push-Off (Right)/1
  Task/1 -> Right Leg Ball/2(Task)
  Right Leg Ball/1(Push-Off Right (Ball)) -> Product1/1
  Product1/1 -> Selector5/1
  Config [5]/1 -> Right Leg Ball/1(Config)
  left/right/1 -> Product1/2, Right Leg Ball/Enable

== system ramadan_2021/Supraspinal Level/Subsystem/Swing Leg/Compute Acceleration Profiles with Minimal Jerk Approach/ Timer Phase 1 ==
  R : Inport
  Clock1 : Clock
  Clock3 : Clock
      settings: Decimation=4
  NOT : Logic  Operator=NOT  AllPortsSameDT=off  OutDataTypeStr=boolean
  Resettable Subsystem : Subsystem  TreatAsAtomicUnit=on
  Sum1 : Sum  Inputs=|+-  InputSameDT=on  SaturateOnIntegerOverflow=on  OutDataTypeStr=Inherit: Same as first input
  Switch2 : Switch  Criteria=u2 > Threshold  RndMeth=Zero
  t_passed : Outport  VectorParamsAs1DForOutWhenUnconnected=off
  wires:
  Clock1/1 -> Sum1/1
  Clock3/1 -> Switch2/3, Resettable Subsystem/1(In1)
  Sum1/1 -> t_passed/1
  R/1 -> NOT/1, Switch2/2
  Switch2/1 -> Sum1/2
  Resettable Subsystem/1(Out1) -> Switch2/1
  NOT/1 -> Resettable Subsystem/Enable

== system ramadan_2021/Supraspinal Level/Subsystem/Swing Leg/Compute Acceleration Profiles with Minimal Jerk Approach/ Timer Phase 2 ==
  R : Inport
  Clock1 : Clock
  Clock3 : Clock
      settings: Decimation=4
  NOT : Logic  Operator=NOT  AllPortsSameDT=off  OutDataTypeStr=boolean
  Resettable Subsystem : Subsystem  TreatAsAtomicUnit=on
  Sum1 : Sum  Inputs=|+-  InputSameDT=on  SaturateOnIntegerOverflow=on  OutDataTypeStr=Inherit: Same as first input
  Switch2 : Switch  Criteria=u2 > Threshold  RndMeth=Zero
  Out : Outport  VectorParamsAs1DForOutWhenUnconnected=off
  wires:
  Clock1/1 -> Sum1/1
  Clock3/1 -> Switch2/3, Resettable Subsystem/1(In1)
  Sum1/1 -> Out/1
  R/1 -> NOT/1, Switch2/2
  Switch2/1 -> Sum1/2
  Resettable Subsystem/1(Out1) -> Switch2/1
  NOT/1 -> Resettable Subsystem/Enable

== system ramadan_2021/Supraspinal Level/Subsystem/Swing Leg/Compute Acceleration Profiles with Minimal Jerk Approach/ Timer Phase 3 ==
  R : Inport
  Clock1 : Clock
  Clock3 : Clock
      settings: Decimation=4
  NOT : Logic  Operator=NOT  AllPortsSameDT=off  OutDataTypeStr=boolean
  Resettable Subsystem : Subsystem  TreatAsAtomicUnit=on
  Sum1 : Sum  Inputs=|+-  InputSameDT=on  SaturateOnIntegerOverflow=on  OutDataTypeStr=Inherit: Same as first input
  Switch2 : Switch  Criteria=u2 > Threshold  RndMeth=Zero
  t_passed : Outport  VectorParamsAs1DForOutWhenUnconnected=off
  wires:
  Clock1/1 -> Sum1/1
  Clock3/1 -> Switch2/3, Resettable Subsystem/1(In1)
  Sum1/1 -> t_passed/1
  R/1 -> NOT/1, Switch2/2
  Switch2/1 -> Sum1/2
  Resettable Subsystem/1(Out1) -> Switch2/1
  NOT/1 -> Resettable Subsystem/Enable

== system ramadan_2021/Supraspinal Level/Subsystem/Swing Leg/Compute Acceleration Profiles with Minimal Jerk Approach/ Timer Phase 4 ==
  R : Inport
  Clock1 : Clock
  Clock3 : Clock
      settings: Decimation=4
  NOT : Logic  Operator=NOT  AllPortsSameDT=off  OutDataTypeStr=boolean
  Resettable Subsystem : Subsystem  TreatAsAtomicUnit=on
  Sum1 : Sum  Inputs=|+-  InputSameDT=on  SaturateOnIntegerOverflow=on  OutDataTypeStr=Inherit: Same as first input
  Switch2 : Switch  Criteria=u2 > Threshold  RndMeth=Zero
  t_passed : Outport  VectorParamsAs1DForOutWhenUnconnected=off
  wires:
  Clock1/1 -> Sum1/1
  Clock3/1 -> Switch2/3, Resettable Subsystem/1(In1)
  Sum1/1 -> t_passed/1
  R/1 -> NOT/1, Switch2/2
  Switch2/1 -> Sum1/2
  Resettable Subsystem/1(Out1) -> Switch2/1
  NOT/1 -> Resettable Subsystem/Enable

== system ramadan_2021/Supraspinal Level/Subsystem/Swing Leg/Compute Acceleration Profiles with Minimal Jerk Approach/Minimal jerk Hip Pitch1 ==
  T_tot : Inport
  t_passed : Inport  Port=2
  "x0, dx0, ddx0" : Inport  Port=3
  "xT, dxT, ddxT" : Inport  Port=4
  Compare To Constant : simulink/Logic and Bit Operations/Compare To Constant  relop=>=  const=mParams.control.timelimit  OutDataTypeStr=boolean  ZeroCross=off
  Constant : Constant  Value=mParams.control.timelimit
  Constant1 : Constant  Value=0
  Demux : Demux  Outputs=3
  Demux1 : Demux  Outputs=3
  Enabled Subsystem : Subsystem  TreatAsAtomicUnit=on
  Minimal Jerk : Subsystem
  Minimal Jerk Parameters [Movellan] : Subsystem
  Minus : Sum  Inputs=+-
  Minus1 : Sum  Inputs=+-
  Switch : Switch
  jerk : Outport
  wires:
  Minimal Jerk/1(j(t)) -> jerk/1
  T_tot/1 -> Minus/1
  t_passed/1 -> Minus/2
  Constant1/1 -> Switch/1
  Demux/1 -> Minimal Jerk Parameters [Movellan]/1(x0)
  Demux/2 -> Minimal Jerk Parameters [Movellan]/2(dx0)
  Demux/3 -> Minimal Jerk Parameters [Movellan]/3(ddx0)
  Demux1/1 -> Minimal Jerk Parameters [Movellan]/4(xT)
  "x0, dx0, ddx0"/1 -> Demux/1
  Demux1/2 -> Minimal Jerk Parameters [Movellan]/5(dxT)
  "xT, dxT, ddxT"/1 -> Demux1/1
  Demux1/3 -> Minimal Jerk Parameters [Movellan]/6(ddxT)
  Minimal Jerk Parameters [Movellan]/1(a) -> Enabled Subsystem/1(In1)
  Minus/1 -> Compare To Constant/1, Minus1/2, Minimal Jerk Parameters [Movellan]/7(T)
  Enabled Subsystem/1(Out1) -> Minimal Jerk/2(a [6x1])
  Compare To Constant/1 -> Switch/2, Enabled Subsystem/Enable
  Constant/1 -> Minus1/1
  Minus1/1 -> Switch/3
  Switch/1 -> Minimal Jerk/1(t)

== system ramadan_2021/Supraspinal Level/Subsystem/Swing Leg/Compute Acceleration Profiles with Minimal Jerk Approach/Minimal jerk Hip Pitch2 ==
  T_tot : Inport
  t_passed : Inport  Port=2
  "x0, dx0, ddx0" : Inport  Port=3
  "xT, dxT, ddxT" : Inport  Port=4
  Compare To Constant : simulink/Logic and Bit Operations/Compare To Constant  relop=>=  const=mParams.control.timelimit  OutDataTypeStr=boolean  ZeroCross=off
  Constant : Constant  Value=mParams.control.timelimit
  Constant1 : Constant  Value=0
  Demux : Demux  Outputs=3
  Demux1 : Demux  Outputs=3
  Enabled Subsystem : Subsystem  TreatAsAtomicUnit=on
  Minimal Jerk : Subsystem
  Minimal Jerk Parameters [Movellan] : Subsystem
  Minus : Sum  Inputs=+-
  Minus1 : Sum  Inputs=+-
  Switch : Switch
  jerk : Outport
  wires:
  Minimal Jerk/1(j(t)) -> jerk/1
  T_tot/1 -> Minus/1
  t_passed/1 -> Minus/2
  Constant1/1 -> Switch/1
  Demux/1 -> Minimal Jerk Parameters [Movellan]/1(x0)
  Demux/2 -> Minimal Jerk Parameters [Movellan]/2(dx0)
  Demux/3 -> Minimal Jerk Parameters [Movellan]/3(ddx0)
  Demux1/1 -> Minimal Jerk Parameters [Movellan]/4(xT)
  "x0, dx0, ddx0"/1 -> Demux/1
  Demux1/2 -> Minimal Jerk Parameters [Movellan]/5(dxT)
  "xT, dxT, ddxT"/1 -> Demux1/1
  Demux1/3 -> Minimal Jerk Parameters [Movellan]/6(ddxT)
  Minimal Jerk Parameters [Movellan]/1(a) -> Enabled Subsystem/1(In1)
  Minus/1 -> Compare To Constant/1, Minus1/2, Minimal Jerk Parameters [Movellan]/7(T)
  Enabled Subsystem/1(Out1) -> Minimal Jerk/2(a [6x1])
  Compare To Constant/1 -> Switch/2, Enabled Subsystem/Enable
  Constant/1 -> Minus1/1
  Minus1/1 -> Switch/3
  Switch/1 -> Minimal Jerk/1(t)

== system ramadan_2021/Supraspinal Level/Subsystem/Swing Leg/Compute Acceleration Profiles with Minimal Jerk Approach/Minimal jerk Hip Pitch3 ==
  T_tot : Inport
  t_passed : Inport  Port=2
  "x0, dx0, ddx0" : Inport  Port=3
  "xT, dxT, ddxT" : Inport  Port=4
  Compare To Constant1 : simulink/Logic and Bit Operations/Compare To Constant  relop=>=  const=mParams.control.timelimit  OutDataTypeStr=boolean  ZeroCross=off
  Constant : Constant  Value=mParams.control.timelimit
  Constant1 : Constant  Value=0
  Demux : Demux  Outputs=3
  Demux1 : Demux  Outputs=3
  Enabled Subsystem : Subsystem  TreatAsAtomicUnit=on
  Minimal Jerk : Subsystem
  Minimal Jerk Parameters [Movellan] : Subsystem
  Minus : Sum  Inputs=+-
  Minus1 : Sum  Inputs=+-
  Switch : Switch
  jerk : Outport
  wires:
  Minimal Jerk/1(j(t)) -> jerk/1
  T_tot/1 -> Minus/1
  t_passed/1 -> Minus/2
  Constant1/1 -> Switch/1
  Demux/1 -> Minimal Jerk Parameters [Movellan]/1(x0)
  Demux/2 -> Minimal Jerk Parameters [Movellan]/2(dx0)
  Demux/3 -> Minimal Jerk Parameters [Movellan]/3(ddx0)
  Demux1/1 -> Minimal Jerk Parameters [Movellan]/4(xT)
  "x0, dx0, ddx0"/1 -> Demux/1
  Demux1/2 -> Minimal Jerk Parameters [Movellan]/5(dxT)
  "xT, dxT, ddxT"/1 -> Demux1/1
  Demux1/3 -> Minimal Jerk Parameters [Movellan]/6(ddxT)
  Minimal Jerk Parameters [Movellan]/1(a) -> Enabled Subsystem/1(In1)
  Minus/1 -> Compare To Constant1/1, Minus1/2, Minimal Jerk Parameters [Movellan]/7(T)
  Enabled Subsystem/1(Out1) -> Minimal Jerk/2(a [6x1])
  Compare To Constant1/1 -> Switch/2, Enabled Subsystem/Enable
  Constant/1 -> Minus1/1
  Minus1/1 -> Switch/3
  Switch/1 -> Minimal Jerk/1(t)

== system ramadan_2021/Supraspinal Level/Subsystem/Swing Leg/Compute Acceleration Profiles with Minimal Jerk Approach/Minimal jerk Hip Pitch4 ==
  T_tot : Inport
  t_passed : Inport  Port=2
  "x0, dx0, ddx0" : Inport  Port=3
  "xT, dxT, ddxT" : Inport  Port=4
  Compare To Constant : simulink/Logic and Bit Operations/Compare To Constant  relop=>=  const=mParams.control.timelimit  OutDataTypeStr=boolean  ZeroCross=off
  Constant : Constant  Value=mParams.control.timelimit
  Constant1 : Constant  Value=0
  Demux : Demux  Outputs=3
  Demux1 : Demux  Outputs=3
  Enabled Subsystem : Subsystem  TreatAsAtomicUnit=on
  Minimal Jerk : Subsystem
  Minimal Jerk Parameters [Movellan] : Subsystem
  Minus : Sum  Inputs=+-
  Minus1 : Sum  Inputs=+-
  Switch : Switch
  jerk : Outport
  wires:
  Minimal Jerk/1(j(t)) -> jerk/1
  T_tot/1 -> Minus/1
  t_passed/1 -> Minus/2
  Constant1/1 -> Switch/1
  Demux/1 -> Minimal Jerk Parameters [Movellan]/1(x0)
  Demux/2 -> Minimal Jerk Parameters [Movellan]/2(dx0)
  Demux/3 -> Minimal Jerk Parameters [Movellan]/3(ddx0)
  Demux1/1 -> Minimal Jerk Parameters [Movellan]/4(xT)
  "x0, dx0, ddx0"/1 -> Demux/1
  Demux1/2 -> Minimal Jerk Parameters [Movellan]/5(dxT)
  "xT, dxT, ddxT"/1 -> Demux1/1
  Demux1/3 -> Minimal Jerk Parameters [Movellan]/6(ddxT)
  Minimal Jerk Parameters [Movellan]/1(a) -> Enabled Subsystem/1(In1)
  Minus/1 -> Compare To Constant/1, Minus1/2, Minimal Jerk Parameters [Movellan]/7(T)
  Enabled Subsystem/1(Out1) -> Minimal Jerk/2(a [6x1])
  Compare To Constant/1 -> Switch/2, Enabled Subsystem/Enable
  Constant/1 -> Minus1/1
  Minus1/1 -> Switch/3
  Switch/1 -> Minimal Jerk/1(t)

== system ramadan_2021/Supraspinal Level/Subsystem/Swing Leg/Compute Acceleration Profiles with Minimal Jerk Approach/Minimal jerk Hip Roll4 ==
  T_tot : Inport
  t_passed : Inport  Port=2
  "x0, dx0, ddx0" : Inport  Port=3
  "xT, dxT, ddxT" : Inport  Port=4
  Constant1 : Constant  Value=0
  Demux : Demux  Outputs=3
  Demux1 : Demux  Outputs=3
  Minimal Jerk : Subsystem
  Minimal Jerk Parameters[Movellan] : Subsystem
  Minus : Sum  Inputs=+-
  Saturation : Saturate  UpperLimit=inf  LowerLimit=0.08
  jerk : Outport
  wires:
  Minimal Jerk/1(j(t)) -> jerk/1
  T_tot/1 -> Minus/1
  Minimal Jerk Parameters[Movellan]/1(a) -> Minimal Jerk/2(a [6x1])
  t_passed/1 -> Minus/2
  Constant1/1 -> Minimal Jerk/1(t)
  Minus/1 -> Saturation/1
  Demux/1 -> Minimal Jerk Parameters[Movellan]/1(x0)
  Demux/2 -> Minimal Jerk Parameters[Movellan]/2(dx0)
  Demux/3 -> Minimal Jerk Parameters[Movellan]/3(ddx0)
  Demux1/1 -> Minimal Jerk Parameters[Movellan]/4(xT)
  "x0, dx0, ddx0"/1 -> Demux/1
  Demux1/2 -> Minimal Jerk Parameters[Movellan]/5(dxT)
  "xT, dxT, ddxT"/1 -> Demux1/1
  Demux1/3 -> Minimal Jerk Parameters[Movellan]/6(ddxT)
  Saturation/1 -> Minimal Jerk Parameters[Movellan]/7(T)

== system ramadan_2021/Supraspinal Level/Subsystem/Swing Leg/Compute Target States/Balance Control lateral ==
  Left/Right : Inport
  Constant : Constant  Value=0
  Constant1 : Constant
  Constant2 : Constant  Value=-1
  Divide : Product  Inputs=**
  Divide1 : Product  Inputs=**
  Minus5 : Sum  Inputs=+++
  Minus6 : Sum  Inputs=+-
  Product : Product
  Selector3 : Selector  InputPortWidth=3  IndexOptions=Index vector (dialog)  Indices=[3]  OutputSizes=1
  Selector4 : Selector  InputPortWidth=3  IndexOptions=Index vector (dialog)  Indices=[3]  OutputSizes=1
  Selector5 : Selector  InputPortWidth=3  IndexOptions=Index vector (dialog)  Indices=[3]  OutputSizes=1
  Switch : Switch  Criteria=u2 > Threshold
  Switch1 : Switch  Criteria=u2 > Threshold
  theta_Hip_swing_target : Outport
  wires:
  Divide/1 -> Minus5/2
  Switch/1 -> Minus6/2
  Divide1/1 -> Minus5/3
  [AnklePosR_rot] -> Selector3/1
  Minus6/1 -> Divide1/1
  Left/Right/1 -> Switch1/2, Switch/2
  [AnklePosL_rot] -> Selector4/1
  [cv_lat] -> Divide/2
  [cd_lat] -> Divide1/2
  Selector4/1 -> Switch/1
  Selector3/1 -> Switch/3
  [CoM_Velocity_rot] -> Selector5/1
  Selector5/1 -> Divide/1
  Constant/1 -> Minus6/1
  Minus5/1 -> theta_Hip_swing_target/1
  Product/1 -> Minus5/1
  [swh_lat] -> Product/2
  Switch1/1 -> Product/1
  Constant1/1 -> Switch1/1
  Constant2/1 -> Switch1/3

== system ramadan_2021/Supraspinal Level/Subsystem/Swing Leg/Compute Target States/Balance Control saggital ==
  Left/Right : Inport
  Early Late : Inport  Port=2
  Constant : Constant  Value=0
  Divide : Product  Inputs=**
  Divide1 : Product  Inputs=**
  Enabled Subsystem : Subsystem  TreatAsAtomicUnit=on
  Minus5 : Sum  Inputs=+++
  Minus6 : Sum  Inputs=+-
  Selector3 : Selector  InputPortWidth=3  IndexOptions=Index vector (dialog)  Indices=[1]  OutputSizes=1
  Selector4 : Selector  InputPortWidth=3  IndexOptions=Index vector (dialog)  Indices=[1]  OutputSizes=1
  Selector5 : Selector  InputPortWidth=3  IndexOptions=Index vector (dialog)  Indices=[1]  OutputSizes=1
  Switch : Switch  Criteria=u2 > Threshold
  theta_Hip_swing_target : Outport
  tag scope: d=global, v_mid=global
  wires:
  [swh] -> Minus5/1
  Switch/1 -> Minus6/2
  [AnklePosR_rot] -> Selector4/1
  Minus6/1 -> [d], Divide1/1
  Left/Right/1 -> Switch/2
  [AnklePosL_rot] -> Selector3/1
  [cv] -> Divide/2
  [cd] -> Divide1/2
  Divide/1 -> Minus5/2
  [CoM_Velocity_rot] -> Selector5/1
  Constant/1 -> Minus6/1
  Divide1/1 -> Minus5/3
  Minus5/1 -> theta_Hip_swing_target/1
  Selector5/1 -> Enabled Subsystem/1(CoM Vel), Divide/1
  Early Late/1 -> Enabled Subsystem/Trigger
  Enabled Subsystem/1(CoM Vel at Midswing) -> [v_mid]
  Selector3/1 -> Switch/1
  Selector4/1 -> Switch/3

== system ramadan_2021/Supraspinal Level/Subsystem/Swing Leg/Inverse Dynamics: Left Leg/Inverse Dynamics ==
  note: Augment Joint Vectors: In order to compute appropriate gravitational and velocity dependend forces, the joint angle and joint angle acceleration vectors are augmented by the position and velocity of the body in space.
  Joint Angles [rad] : Inport
  Joint Angle Velocities [rad/s] : Inport  Port=2
  Joint  Acceleration [rad/s^2] : Inport  Port=3
  Rotation Trunk [rad] : Inport  Port=4
  Trunk Position [m] : Inport  Port=5
  Rotation Velocity Trunk [rad/s] : Inport  Port=6
  Trunk Velocity [m/s] : Inport  Port=7
  Desired Acceleration [rad/s^2] : Inport  Port=8
  Enable : EnablePort  ZeroCross=off
  Constant : Constant  Value=zeros(6,1)
  Inverse Dynamics : Subsystem
  Mux : Mux  Inputs=3
  Mux1 : Mux  Inputs=3
  Mux2 : Mux  Inputs=2
  Mux4 : Mux  Inputs=2
  " Desired Torques" : Outport  VectorParamsAs1DForOutWhenUnconnected=off
  Interaction Wrench : Outport  Port=2  VectorParamsAs1DForOutWhenUnconnected=off
  wires:
  Trunk Position [m]/1 -> Mux1/1
  Inverse Dynamics/1(Desired Torques) -> " Desired Torques"/1
  Mux1/1 -> Inverse Dynamics/1(Config)
  Joint Angles [rad]/1 -> Mux1/3
  Rotation Trunk [rad]/1 -> Mux1/2
  Joint Angle Velocities [rad/s]/1 -> Mux/3
  Mux/1 -> Inverse Dynamics/2(JointVel)
  Desired Acceleration [rad/s^2]/1 -> Mux2/2
  Mux2/1 -> Inverse Dynamics/3(Des. JointAccel)
  Inverse Dynamics/2(Interaction Wrench Left) -> Interaction Wrench/1
  Constant/1 -> Mux4/1, Mux2/1
  Mux4/1 -> Inverse Dynamics/4(Real JointAccel)
  Joint  Acceleration [rad/s^2]/1 -> Mux4/2
  Trunk Velocity [m/s]/1 -> Mux/1
  Rotation Velocity Trunk [rad/s]/1 -> Mux/2

== system ramadan_2021/Supraspinal Level/Subsystem/Swing Leg/Inverse Dynamics: Left Leg/Sensor Data from Body Layer ==
  Constant : Constant  Commented=on  Value=0
  Constant1 : Constant  Value=zeros(3,1)
  From3 : From  Commented=on  GotoTag=TrunkRot_lat  TagVisibility=global
  From4 : From  Commented=on  GotoTag=TrunkRot_sag  TagVisibility=global
  From44 : From  Commented=on  GotoTag=RotationalVelocityTrunk  TagVisibility=global
  From46 : From  Commented=on  GotoTag=TranslationalVelocityTrunk  TagVisibility=global
  Gain : Gain  Gain=0
  Gain1 : Gain  Gain=0
  Mux : Mux  Commented=on  Inputs=3
  Sensor Delay 1 : eeGeneralControl/Low-Pass Filter (Discrete or Continuous)  K=1  T=0.01  B=inf  A=-inf  init_option=Inherited from block input  x0=0  Ts=0
  Sensor Delay 2 : eeGeneralControl/Low-Pass Filter (Discrete or Continuous)  K=1  T=0.01  B=inf  A=-inf  init_option=Inherited from block input  x0=0  Ts=0
  Sensor Delay 3 : eeGeneralControl/Low-Pass Filter (Discrete or Continuous)  K=1  T=0.01  B=inf  A=-inf  init_option=Inherited from block input  x0=0  Ts=0
  Joint Angles [rad] : Outport
  Joint Angle Velocities [rad/s] : Outport  Port=2
  Joint Angle Accelerations [rad/s^2] : Outport  Port=3
  " Rotation Trunk [rad]" : Outport  Port=4
  Trunk Position [m] : Outport  Port=5
  Rotation Velocity Trunk [rad/s] : Outport  Port=6
  Trunk Velocity [m/s] : Outport  Port=7
  wires:
  [Llegq] -> Sensor Delay 3/1
  [Llegdq] -> Sensor Delay 1/1
  Sensor Delay 3/1 -> Joint Angles [rad]/1
  Sensor Delay 1/1 -> Joint Angle Velocities [rad/s]/1
  [CoM_Position] -> Trunk Position [m]/1
  [Llegddq] -> Sensor Delay 2/1
  Sensor Delay 2/1 -> Joint Angle Accelerations [rad/s^2]/1
  From3/1 -> Mux/1
  Constant/1 -> Mux/2
  From4/1 -> Mux/3
  [RotationTrunk] -> " Rotation Trunk [rad]"/1
  Gain/1 -> Rotation Velocity Trunk [rad/s]/1
  Gain1/1 -> Trunk Velocity [m/s]/1
  Constant1/1 -> Gain1/1, Gain/1

== system ramadan_2021/Supraspinal Level/Subsystem/Swing Leg/Inverse Dynamics: Right Leg/Inverse Dynamics1 ==
  note: Augment Joint Vectors: In order to compute appropriate gravitational and velocity dependend forces, the joint angle and joint angle acceleration vectors are augmented by the position and velocity of the body in space.
  Joint Angles [rad] : Inport
  Joint Angle Velocities [rad/s] : Inport  Port=2
  Joint  Acceleration [rad/s^2] : Inport  Port=3
  Rotation Trunk [rad] : Inport  Port=4
  Trunk Position [m] : Inport  Port=5
  Rotation Velocity Trunk [rad/s] : Inport  Port=6
  Trunk Velocity [m/s] : Inport  Port=7
  Desired Acceleration [rad/s^2] : Inport  Port=8
  Enable : EnablePort  ZeroCross=off
  Constant : Constant  Value=zeros(6,1)
  Inverse Dynamics : Subsystem
  Mux : Mux  Inputs=3
  Mux1 : Mux  Inputs=3
  Mux2 : Mux  Inputs=2
  Mux4 : Mux  Inputs=2
  " Desired Torques" : Outport  VectorParamsAs1DForOutWhenUnconnected=off
  Interaction Wrench : Outport  Port=2  VectorParamsAs1DForOutWhenUnconnected=off
  wires:
  Trunk Position [m]/1 -> Mux1/1
  Inverse Dynamics/1(Desired Torques) -> " Desired Torques"/1
  Mux1/1 -> Inverse Dynamics/1(Config)
  Joint Angles [rad]/1 -> Mux1/3
  Rotation Trunk [rad]/1 -> Mux1/2
  Joint Angle Velocities [rad/s]/1 -> Mux/3
  Mux/1 -> Inverse Dynamics/2(JointVel)
  Desired Acceleration [rad/s^2]/1 -> Mux2/2
  Mux2/1 -> Inverse Dynamics/3(Des. JointAccel)
  Constant/1 -> Mux4/1, Mux2/1
  Mux4/1 -> Inverse Dynamics/4(Real JointAccel)
  Joint  Acceleration [rad/s^2]/1 -> Mux4/2
  Inverse Dynamics/2(Interaction Wrench Left) -> Interaction Wrench/1
  Trunk Velocity [m/s]/1 -> Mux/1
  Rotation Velocity Trunk [rad/s]/1 -> Mux/2
